simulink model "FIR_SymmetricDecimatorStream_Ex2"  (R2023a)
settings: Solver=VariableStepAuto  StartTime=0.0  StopTime=1  RelTol=1e-3
PostLoadFcn:
  | Fs = 100000;  % Sampling Frequency
  | Fpass = 5000;              % Passband Frequency
  | Fstop = 10000;             % Stopband Frequency
  | Dpass = 0.0046051376314;   % Passband Ripple
  | Dstop = 0.00025118864315;  % Stopband Attenuation
  | dens  = 16;                % Density Factor
  | % Calculate the order from the parameters using FIRPMORD.
  | [N, Fo, Ao, W] = firpmord([Fpass, Fstop]/(Fs/2), [1 0], [Dpass, Dstop]);
  | % Calculate the coefficients using the FIRPM function.
  | coeffs = firpm(N, Fo, Ao, W, {dens});
  | AIE_Coeffs = (int16(coeffs(1:32)*2^15));
undefined symbols (not defined in the file): firpmord, None, S, vsva2197, xcvc1902
libraries: aieUtilities x4, aieDSP x1, dspsrcs4 x1, dspmlti4 x1, vmcUtilities x1
settings Model: Creator=sdegala  LastModifiedBy=robg
settings ModelReferenceCC: EnableRefExpFcnMdlSchedulingChecks=on

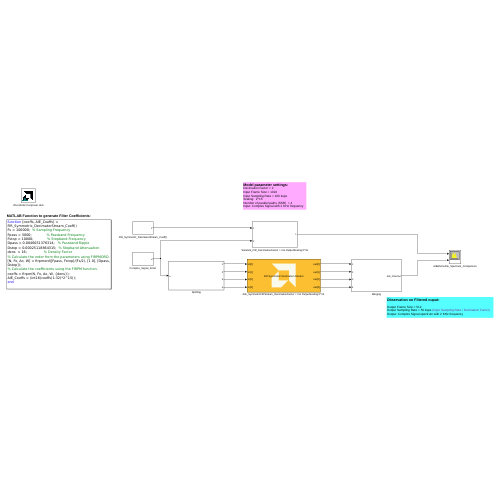
[thumbnail: Simulink's stored preview of the top-level diagram]
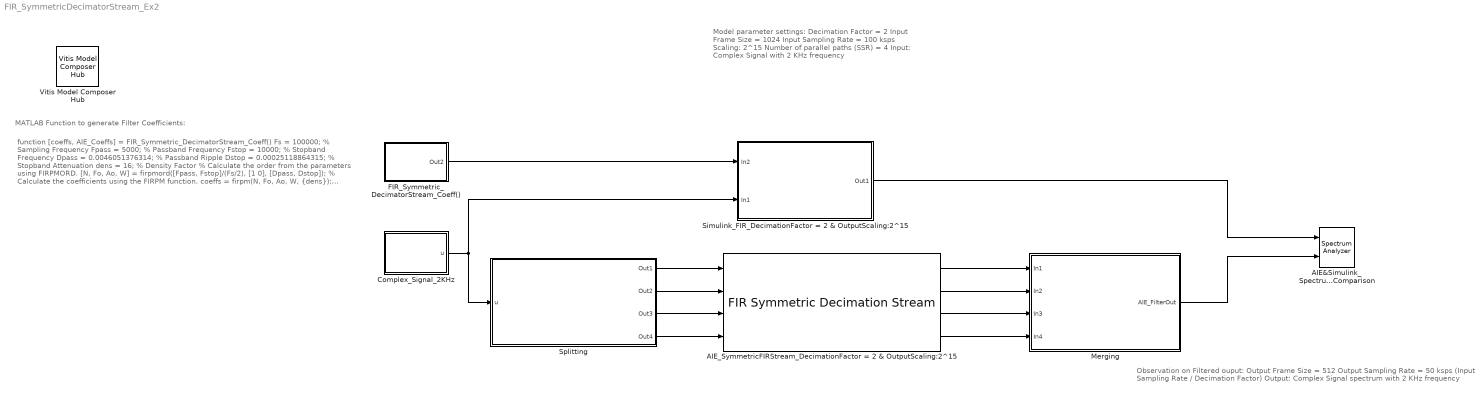
== system FIR_SymmetricDecimatorStream_Ex2 ==
  note: Model parameter settings:
      | Decimation Factor = 2
      | Input Frame Size = 1024
      | Input Sampling Rate = 100 ksps
      | Scaling: 2^15
      | Number of parallel paths (SSR) = 4
      | Input: Complex Signal with 2 KHz frequency
  note: Observation on Filtered ouput:
      |
      | Output Frame Size = 512
      | Output Sampling Rate = 50 ksps (Input Sampling Rate / Decimation Factor)
      | Output: Complex Signal spectrum with 2 KHz frequency
  note: function [coeffs, AIE_Coeffs] = FIR_Symmetric_DecimatorStream_Coeff()
      | Fs = 100000; % Sampling Frequency
      | Fpass = 5000; % Passband Frequency
      | Fstop = 10000; % Stopband Frequency
      | Dpass = 0.0046051376314; % Passband Ripple
      | Dstop = 0.00025118864315; % Stopband Attenuation
      | dens = 16; % Density Factor
      | % Calculate the order from the parameters using FIRPMORD.
      | [N, Fo, Ao, W] = firpmord([Fpass, Fstop]/(Fs/2), [1 0], [Dpass, Dstop]);
      | % Calculate the coefficients using the FIRPM function.
      | coeffs = firpm(N, Fo, Ao, W, {dens});
      | AIE_Coeffs = (int16(coeffs(1:32)*2^15));
      | end
  note: MATLAB Function to generate Filter Coefficients:
  AIE&Simulink_Spectrum_Comparison : SpectrumAnalyzer  NumInputPorts=2  AveragingMethod=Exponential  ShowLegend=on  ChannelNames="[\"\"]"  DefaultConfigurationName=spbscopes.SpectrumAnalyzerBlockCfg
  "AIE_SymmetricFIRStream_DecimationFactor = 2 & OutputScaling:2^15 " : aieDSP/FIR Symmetric Decimation Stream  data_type=cint16  coef_type=int16  use_coeff_reload=off  dual_ip=off  num_outputs=off  coeff=AIE_Coeffs  fir_length=64  decimate_factor=2  input_window_size=1024  shift_val=15  rnd_mode=Ceiling  sat_mode=0-None  ssr=4  casc_length=1  AIE_VARIANT=1  blockJsonConstraints=[]  blockJsonConstraintsInternal=[]  spec=vmc_stream_fir_decimate_sym.json  SerializedMaskParamNames=[]  SerializedMaskParamValues=[]  SerializedMaskParamVisibilities=[]  block_type=FIR Symmetric Decimation Stream  SerializedMaskParamDataypes=typename|typename|bool|bool|bool|coef_type|uint|uint|uint|uint|uint|uint|uint|uint|uint  SerializedMaskParamEnumStrArr=0|0|0|0|0|0|0|0|0|0|Floor,Ceiling,Round to positive infinity,Round to negative infinity,Round symmetrical to infinity,Round symmetrical to zero,Round convergent to even,Round convergent to odd|0-None,1-Asymmetric,3-Symmetric|0|0|0  SerializedMaskParamEnumValArr=0|0|0|0|0|0|0|0|0|0|0,1,2,3,4,5,6,7|0,1,3|0|0|0  SerializedMaskParamVectorArr=0|0|0|0|0|1|0|0|0|0|0|0|0|0|0
  Complex_Signal_2KHz : Subsystem
  FIR_Symmetric_DecimatorStream_Coeff() : Subsystem
  Merging : Subsystem
  Simulink_FIR_DecimationFactor = 2 & OutputScaling:2^15 : Subsystem
  Splitting : Subsystem
  Vitis Model Composer Hub : vmcUtilities/Vitis Model Composer Hub  Tag=genX  CodeGeneration=off  StartColumn=1  NumberOfColumns=1  TargetDirectory=./code  exportDesign=off  analyzeDesign=off  validateDesignOnHw=off  ExportType=AI Engines  IpVendor=xilinx.com  IpLibrary=hls  IpVersion=1.0  IpHWLanguage=Verilog  AieCompilerOptions={}  AieSimulatorOptions={}  CreateTestbench=off  TestbenchStackSize=10  RunRtlSim=off  RunCSim=off  RunAieSim=off  AieSimTimeout=50000  RunAieSimProfiling=off  LaunchVitisAnalyzer=off  PlotOutput=off  RunX86Sim=off  X86SimTimeout=10  GenHwImage=off  GenLibadfXo=off  GenHwValidationCode=off  PlatformType=Not Specified  HwSystemType=Baremetal  HwValidationTarget=hw  ProjDevice=xcvc1902-vsva2197-1LP-e-S  ProjDevicePart=xcvc1902-vsva2197-1LP-e-S  AIEType=AIE  SamplePeriod=-1  ClockFrequency=200  DataPathParallelism=1  xilinxfamily=versalaicore  part=xcvc1902  speed=-1LP-e-S  package=vsva2197  directory=./netlist  testbench=off  incr_netlist=off  synthesis_tool=Vivado  clock_wrapper=Clock Enables  dbl_ovrd=According to Block Masks  dcm_input_clock_period=10  sysclk_period=10  simulink_period=1  eval_field=0  LogFileName=''  NThreads=4
  wires:
  Splitting/1(Out1) -> "AIE_SymmetricFIRStream_DecimationFactor = 2 & OutputScaling:2^15 "/1
  Splitting/2(Out2) -> "AIE_SymmetricFIRStream_DecimationFactor = 2 & OutputScaling:2^15 "/2
  Splitting/3(Out3) -> "AIE_SymmetricFIRStream_DecimationFactor = 2 & OutputScaling:2^15 "/3
  Splitting/4(Out4) -> "AIE_SymmetricFIRStream_DecimationFactor = 2 & OutputScaling:2^15 "/4
  "AIE_SymmetricFIRStream_DecimationFactor = 2 & OutputScaling:2^15 "/1 -> Merging/1(In1)
  "AIE_SymmetricFIRStream_DecimationFactor = 2 & OutputScaling:2^15 "/2 -> Merging/2(In2)
  "AIE_SymmetricFIRStream_DecimationFactor = 2 & OutputScaling:2^15 "/3 -> Merging/3(In3)
  "AIE_SymmetricFIRStream_DecimationFactor = 2 & OutputScaling:2^15 "/4 -> Merging/4(In4)
  FIR_Symmetric_DecimatorStream_Coeff()/1(Out2) -> Simulink_FIR_DecimationFactor = 2 & OutputScaling:2^15/1(In2)
  Complex_Signal_2KHz/1(u) -> Simulink_FIR_DecimationFactor = 2 & OutputScaling:2^15/2(In1), Splitting/1(u)
  Merging/1(AIE_FilterOut) -> AIE&Simulink_Spectrum_Comparison/2
  Simulink_FIR_DecimationFactor = 2 & OutputScaling:2^15/1(Out1) -> AIE&Simulink_Spectrum_Comparison/1

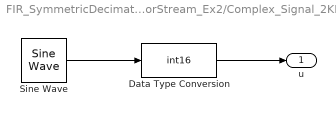
== system FIR_SymmetricDecimatorStream_Ex2/Complex_Signal_2KHz ==
  Data Type Conversion : DataTypeConversion  OutMin=[-1]  OutMax=[1]  OutDataTypeStr=int16  ConvertRealWorld=Stored Integer (SI)  SaturateOnIntegerOverflow=off  RndMeth=Floor
  Sine Wave : dspsrcs4/Sine Wave  Amplitude=1  Frequency=2e3  Phase=0  SampleMode=Discrete  OutComplex=Complex  CompMethod=Table lookup  TableSize=Speed  SampleTime=1/100e3  SamplesPerFrame=1024  ResetState=Restart at time zero  OutputFrames=off  dataType=Fixed-point  wordLen=16  udDataType=sfix(16)  fracBitsMode=User-defined  numFracBits=14  OutDataTypeStr=fixdt(1,16,14)  LastOutDataTypeStr=fixdt(1,16,14)
  u : Outport
  wires:
  Sine Wave/1 -> Data Type Conversion/1
  Data Type Conversion/1 -> u/1

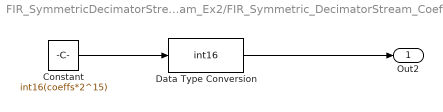
== system FIR_SymmetricDecimatorStream_Ex2/FIR_Symmetric_DecimatorStream_Coeff() ==
  Constant : Constant  Value=int16(coeffs*2^15)
  Data Type Conversion : DataTypeConversion  OutMin=[-1]  OutMax=[1]  OutDataTypeStr=int16  ConvertRealWorld=Stored Integer (SI)  SaturateOnIntegerOverflow=off  RndMeth=Floor
  Out2 : Outport
  wires:
  Constant/1 -> Data Type Conversion/1
  Data Type Conversion/1 -> Out2/1

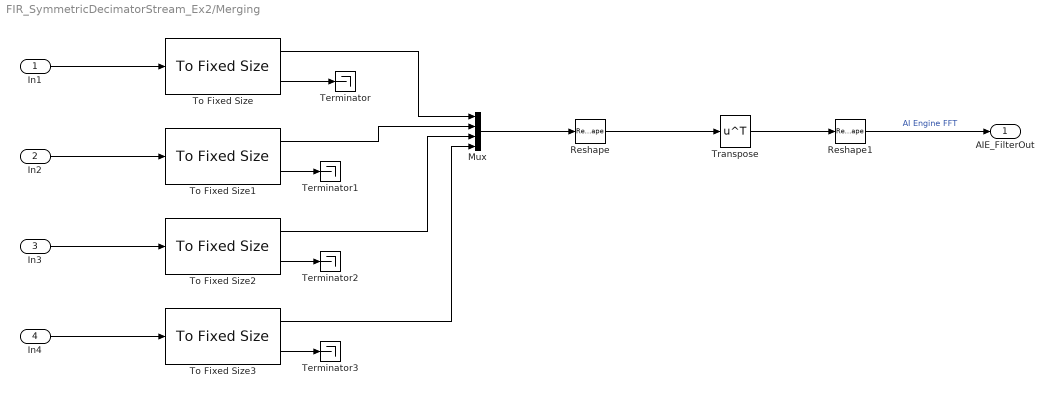
== system FIR_SymmetricDecimatorStream_Ex2/Merging ==
  In1 : Inport
  In2 : Inport  Port=2
  In3 : Inport  Port=3
  In4 : Inport  Port=4
  Mux : Mux
  Reshape : Reshape  OutputDimensionality=Customize  OutputDimensions=[128, 4]
  Reshape1 : Reshape  OutputDimensions=[1, 10]
  Terminator{,1..3} (4 alike) : Terminator
  To Fixed Size{,1..3} (4 alike) : aieUtilities/To Fixed Size  Mode=Produce a valid output signal  OutputSize=Inherit: Same as input  CopyMethod=Buffer samples to form output  HasStatusOutput=on
  Transpose : Math  Operator=transpose
  AIE_FilterOut : Outport
  wires:
  Reshape/1 -> Transpose/1
  To Fixed Size1/2 -> Terminator1/1
  To Fixed Size1/1 -> Mux/2
  In2/1 -> To Fixed Size1/1
  To Fixed Size/2 -> Terminator/1
  Transpose/1 -> Reshape1/1
  To Fixed Size/1 -> Mux/1
  Mux/1 -> Reshape/1
  Reshape1/1 -> AIE_FilterOut/1  "AI Engine FFT"
  In1/1 -> To Fixed Size/1
  To Fixed Size2/2 -> Terminator2/1
  In4/1 -> To Fixed Size3/1
  To Fixed Size3/1 -> Mux/4
  To Fixed Size3/2 -> Terminator3/1
  In3/1 -> To Fixed Size2/1
  To Fixed Size2/1 -> Mux/3

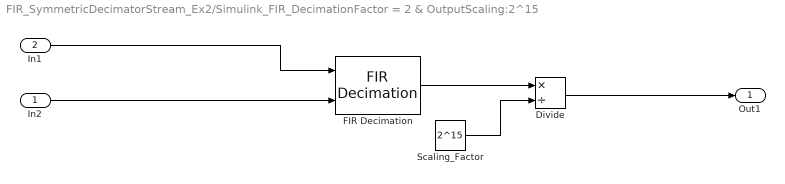
== system FIR_SymmetricDecimatorStream_Ex2/Simulink_FIR_DecimationFactor = 2 & OutputScaling:2^15 ==
  In2 : Inport
  In1 : Inport  Port=2
  Divide : Product  Inputs=*/  OutDataTypeStr=int16
  FIR Decimation : dspmlti4/FIR Decimation  FilterSource=Input port  h=int16(firpm(63, [0;0.1;0.2;1], [1;1;0;0], [1;18.3333831245308], {16})*2^15)  D=2  filtStruct=Direct form  FilterObject=firpmord([5e3, 10e3]/(100e3/2), [1 0], [0.0046051376314, 0.0001995262315])  InputProcessing=Columns as channels (frame based)  framing=Enforce single-rate processing  AllowArbitraryInputLength=off  inputOffset=0  outputBufInitCond=0  roundingMode=Floor  overflowMode=off  firstCoeffDataTypeStr=Inherit: Same word length as input  firstCoeffMin=[]  firstCoeffMax=[]  firstCoeffLastDataTypeStr=Inherit: Same word length as input  prodOutputMode=Binary point scaling  prodOutputWordLength=32  prodOutputFracLength=0  prodOutputDataTypeStr=fixdt(1,32,0)  prodOutputLastDataTypeStr=fixdt(1,32,0)  accumMode=Binary point scaling  accumWordLength=48  accumFracLength=0  accumDataTypeStr=fixdt(1,48,0)  accumLastDataTypeStr=fixdt(1,48,0)  outputDataTypeStr=Inherit: Same as product output  outputMin=[]  outputMax=[]  outputLastDataTypeStr=Inherit: Same as product output
  Scaling_Factor : Constant  Value=2^15  OutDataTypeStr=int32
  Out1 : Outport
  wires:
  Scaling_Factor/1 -> Divide/2
  FIR Decimation/1 -> Divide/1
  In1/1 -> FIR Decimation/1
  Divide/1 -> Out1/1
  In2/1 -> FIR Decimation/2

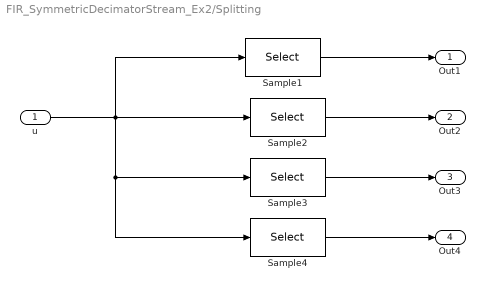
== system FIR_SymmetricDecimatorStream_Ex2/Splitting ==
  u : Inport
  Sample1 : Selector  InputPortWidth=1024  IndexOptions=Index vector (dialog)  Indices=1:4:1024  OutputSizes=1
  Sample2 : Selector  InputPortWidth=1024  IndexOptions=Index vector (dialog)  Indices=2:4:1024  OutputSizes=1
  Sample3 : Selector  InputPortWidth=1024  IndexOptions=Index vector (dialog)  Indices=3:4:1024  OutputSizes=1
  Sample4 : Selector  InputPortWidth=1024  IndexOptions=Index vector (dialog)  Indices=4:4:1024  OutputSizes=1
  Out1 : Outport
  Out2 : Outport  Port=2
  Out3 : Outport  Port=3
  Out4 : Outport  Port=4
  wires:
  u/1 -> Sample4/1, Sample3/1, Sample2/1, Sample1/1
  Sample2/1 -> Out2/1
  Sample1/1 -> Out1/1
  Sample3/1 -> Out3/1
  Sample4/1 -> Out4/1
